simulink library "Energy_Consumption"  (R2018b)
settings: Solver=VariableStepAuto  StartTime=0.0  StopTime=10.0  RelTol=1e-3
values from neighbouring files (symbols this model uses):
  D_v = 0.2*exp(-3)    [glob.m]
  Jp = 4.1904.*exp(-5 )    [glob.m]
  k_t = 0.0104.*exp(-3)    [glob.m]
  k_v = 96.342    [glob.m]
settings Model: Creator=Andrew Garcia  LastModifiedBy=Andrew Garcia

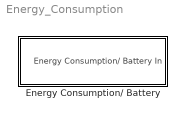
== system Energy_Consumption ==
  Energy Consumption/ Battery : Subsystem  LoadFcn=glob  InitFcn=glob

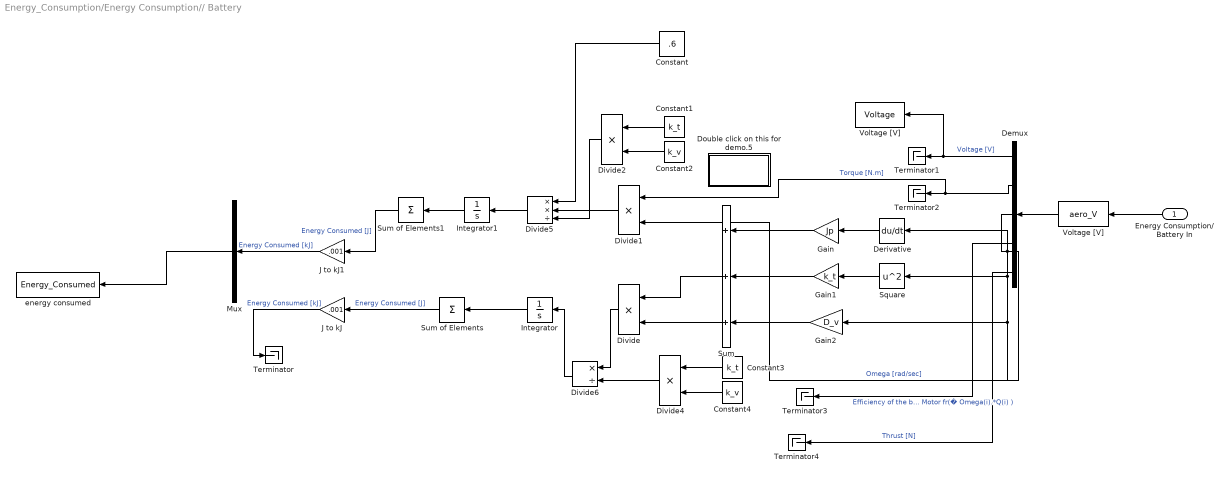
== system Energy_Consumption/Energy Consumption// Battery ==
  Energy Consumption/ Battery In : Inport
  Constant : Constant  Value=.6
  Constant1 : Constant  Value=k_t
  Constant2 : Constant  Value=k_v
  Constant3 : Constant  Value=k_t
  Constant4 : Constant  Value=k_v
  Demux : Demux  Outputs=5
  Derivative : Derivative
  Divide{,1..2,4} (4 alike) : Product  Inputs=**
  Divide5 : Product  Inputs=**/
  Divide6 : Product  Inputs=*/
  Double click on this for demo.5 : Subsystem
      settings: OpenFcn=glob
      mask Display: disp('optsiminit')
  Gain : Gain  Gain=Jp
  Gain1 : Gain  Gain=k_t
  Gain2 : Gain  Gain=D_v
  Integrator : Integrator
  Integrator1 : Integrator
  J to kJ : Gain  Gain=.001
  J to kJ1 : Gain  Gain=.001
  Mux : Mux  Inputs=1
  Square : Math  Operator=square  SaturateOnIntegerOverflow=on
  Sum : Sum  Inputs=+++
  Sum of Elements : Sum  Inputs=+
  Sum of Elements1 : Sum  Inputs=+
  Terminator{,1..4} (5 alike) : Terminator
  Voltage [V] : ToWorkspace  VariableName=Voltage  SampleTime=-1
  "Voltage [V] " : MATLABFcn  MATLABFcn=aero_V  OutputDimensions=20  OutputSignalType=real
  energy consumed : ToWorkspace  VariableName=Energy_Consumed  SampleTime=-1
  wires:
  Constant/1 -> Divide5/1
  Divide/1 -> Divide6/1
  Constant4/1 -> Divide4/2
  Divide4/1 -> Divide6/2
  Constant3/1 -> Divide4/1
  Constant2/1 -> Divide2/2
  Constant1/1 -> Divide2/1
  Divide2/1 -> Divide5/3
  Divide5/1 -> Integrator1/1
  Divide6/1 -> Integrator/1
  Demux/5 -> Terminator4/1  "Thrust [N]"
  J to kJ1/1 -> Mux/1  "Energy Consumed [kJ]"
  Sum of Elements1/1 -> J to kJ1/1  "Energy Consumed [J]"
  Divide1/1 -> Divide5/2
  Integrator1/1 -> Sum of Elements1/1
  Mux/1 -> energy consumed/1
  Demux/4 -> Terminator3/1  "Efficiency of the brushless DC Motor fr(� Omega(i).*Q(i) )"
  Demux/1 -> Terminator1/1, Voltage [V]/1  "Voltage [V]"
  Demux/2 -> Terminator2/1, Divide1/1  "Torque [N.m]"
  J to kJ/1 -> Terminator/1  "Energy Consumed [kJ]"
  Sum of Elements/1 -> J to kJ/1  "Energy Consumed [J]"
  Integrator/1 -> Sum of Elements/1
  Sum/1 -> Divide/1
  Gain2/1 -> Sum/3
  Gain1/1 -> Sum/2
  Gain/1 -> Sum/1
  Square/1 -> Gain1/1
  Derivative/1 -> Gain/1
  Demux/3 -> Square/1, Gain2/1, Divide/2, Derivative/1, Divide1/2  "Omega [rad/sec]"
  "Voltage [V] "/1 -> Demux/1
  Energy Consumption/ Battery In/1 -> "Voltage [V] "/1

== system Energy_Consumption/Energy Consumption// Battery/Double click on this for demo.5 ==
